simulink model "RmtAPP_DD1"  (R2016b)
settings: configuration reference "CodeGenConfigSet" (kept outside this file)
values from neighbouring files (symbols this model uses):
  RmtAPP_tiSRCHighDefDeb_C = Calibration.Parameter    [init_RmtAPP_DD1.m]    (also in init_RmtAPP_DD1_SIL.m = Simulink.Parameter)
  RmtAPP_tiSRCHighOKDeb_C = Calibration.Parameter    [init_RmtAPP_DD1.m]    (also in init_RmtAPP_DD1_SIL.m = Simulink.Parameter)
  RmtAPP_tiSRCLowDefDeb_C = Calibration.Parameter    [init_RmtAPP_DD1.m]    (also in init_RmtAPP_DD1_SIL.m = Simulink.Parameter)
  RmtAPP_tiSRCLowOKDeb_C = Calibration.Parameter    [init_RmtAPP_DD1.m]    (also in init_RmtAPP_DD1_SIL.m = Simulink.Parameter)
  RmtAPP_uRaw1Def_C = Calibration.Parameter    [init_RmtAPP_DD1.m]    (also in init_RmtAPP_DD1_SIL.m = Simulink.Parameter)
  RmtAPP_uRaw1SRCHigh_C = Calibration.Parameter    [init_RmtAPP_DD1.m]    (also in init_RmtAPP_DD1_SIL.m = Simulink.Parameter)
  RmtAPP_uRaw1SRCLow_C = Calibration.Parameter    [init_RmtAPP_DD1.m]    (also in init_RmtAPP_DD1_SIL.m = Simulink.Parameter)
undefined symbols (not defined in the file or in its folder): RmtAPP_DD1_DT
libraries: CXLib x6
settings Model: Creator=bianxuyin  LastModifiedBy=bianxuyin
settings ConfigSetRef: SourceLocation=Base Workspace

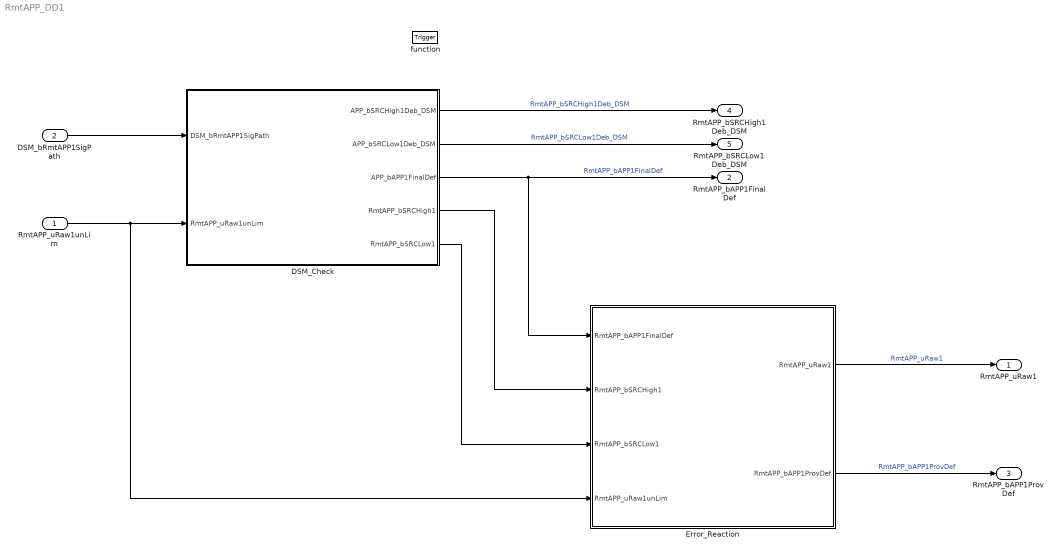
== system RmtAPP_DD1 ==
  RmtAPP_uRaw1unLim : Inport  Tag=mv  Description=Remote Acceleration pedal sensor 1 unlimited raw value  OutMin=0  OutMax=5000  OutDataTypeStr=Ad_mv
  DSM_bRmtAPP1SigPath : Inport  Description=status of FId_RmtAPP1SigPath  Port=2  OutMin=0  OutMax=1  OutDataTypeStr=boolean
  function : TriggerPort  TriggerType=function-call  VariantControl=Variant
  DSM_Check : Subsystem
  Error_Reaction : Subsystem
  RmtAPP_uRaw1 : Outport  Tag=mv  Description=Remote Acceleration Pedal Position D  OutMin=0  OutMax=5000  OutDataTypeStr=Ad_mv
  RmtAPP_bAPP1FinalDef : Outport  Description=Status Sensor 1 of the remote acceleration pedal finally defect  Port=2  OutMin=0  OutMax=1  OutDataTypeStr=boolean
  RmtAPP_bAPP1ProvDef : Outport  Description=Status Sensor 1 of the remote acceleration pedal temporary defect  Port=3  OutMin=0  OutMax=1  OutDataTypeStr=boolean
  RmtAPP_bSRCHigh1Deb_DSM : Outport  Description=Status debounced SRC-High error Sensor 1  Port=4  OutMin=0  OutMax=1  OutDataTypeStr=boolean
  RmtAPP_bSRCLow1Deb_DSM : Outport  Description=Status debounced SRC-Low error Sensor 1  Port=5  OutMin=0  OutMax=1  OutDataTypeStr=boolean
  wires:
  Error_Reaction/1(RmtAPP_uRaw1) -> RmtAPP_uRaw1/1  "RmtAPP_uRaw1"
  DSM_Check/3(APP_bAPP1FinalDef) -> Error_Reaction/1(RmtAPP_bAPP1FinalDef), RmtAPP_bAPP1FinalDef/1  "RmtAPP_bAPP1FinalDef"
  Error_Reaction/2(RmtAPP_bAPP1ProvDef) -> RmtAPP_bAPP1ProvDef/1  "RmtAPP_bAPP1ProvDef"
  DSM_Check/1(APP_bSRCHigh1Deb_DSM) -> RmtAPP_bSRCHigh1Deb_DSM/1  "RmtAPP_bSRCHigh1Deb_DSM"
  DSM_Check/2(APP_bSRCLow1Deb_DSM) -> RmtAPP_bSRCLow1Deb_DSM/1  "RmtAPP_bSRCLow1Deb_DSM"
  RmtAPP_uRaw1unLim/1 -> DSM_Check/2(RmtAPP_uRaw1unLim), Error_Reaction/4(RmtAPP_uRaw1unLim)
  DSM_bRmtAPP1SigPath/1 -> DSM_Check/1(DSM_bRmtAPP1SigPath)
  DSM_Check/4(RmtAPP_bSRCHigh1) -> Error_Reaction/2(RmtAPP_bSRCHigh1)
  DSM_Check/5(RmtAPP_bSRCLow1) -> Error_Reaction/3(RmtAPP_bSRCLow1)

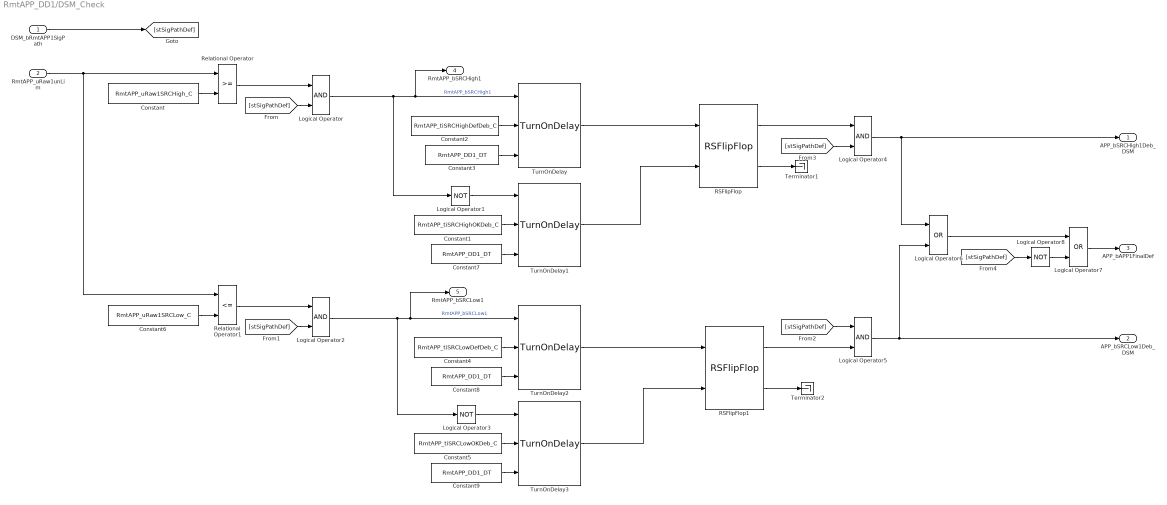
== system RmtAPP_DD1/DSM_Check ==
  DSM_bRmtAPP1SigPath : Inport  Description=status of FId_RmtAPP1SigPath  OutMin=0  OutMax=1  OutDataTypeStr=boolean
  RmtAPP_uRaw1unLim : Inport  Tag=mv  Description=Remote Acceleration pedal sensor 1 unlimited raw value  Port=2  OutMin=0  OutMax=5000  OutDataTypeStr=Ad_mv
  Constant : Constant  Value=RmtAPP_uRaw1SRCHigh_C
  Constant1 : Constant  Value=RmtAPP_tiSRCHighOKDeb_C
  Constant2 : Constant  Value=RmtAPP_tiSRCHighDefDeb_C
  Constant{3,7..9} (4 alike) : Constant  Value=RmtAPP_DD1_DT  OutDataTypeStr=Inherit: Inherit via back propagation
  Constant4 : Constant  Value=RmtAPP_tiSRCLowDefDeb_C
  Constant5 : Constant  Value=RmtAPP_tiSRCLowOKDeb_C
  Constant6 : Constant  Value=RmtAPP_uRaw1SRCLow_C
  Logical Operator{,2,4..5} (4 alike) : Logic  AllPortsSameDT=off  OutDataTypeStr=boolean
  Logical Operator1 : Logic  Operator=NOT  AllPortsSameDT=off  OutDataTypeStr=boolean
  Logical Operator3 : Logic  Operator=NOT  AllPortsSameDT=off  OutDataTypeStr=boolean
  Logical Operator6 : Logic  Operator=OR  AllPortsSameDT=off  OutDataTypeStr=boolean
  Logical Operator7 : Logic  Operator=OR  AllPortsSameDT=off  OutDataTypeStr=boolean
  Logical Operator8 : Logic  Operator=NOT  AllPortsSameDT=off  OutDataTypeStr=boolean
  RSFlipFlop : CXLib/RSFlipFlop
  RSFlipFlop1 : CXLib/RSFlipFlop
  Relational Operator : RelationalOperator  OutDataTypeStr=boolean  RndMeth=Simplest
  Relational Operator1 : RelationalOperator  Operator=<=  OutDataTypeStr=boolean  RndMeth=Simplest
  Terminator1 : Terminator
  Terminator2 : Terminator
  TurnOnDelay{,1..3} (4 alike) : CXLib/TurnOnDelay
  APP_bSRCHigh1Deb_DSM : Outport  Description=Status debounced SRC-High error Sensor 1  OutMin=0  OutMax=1  OutDataTypeStr=boolean
  APP_bSRCLow1Deb_DSM : Outport  Description=Status debounced SRC-Low error Sensor 1  Port=2  OutMin=0  OutMax=1  OutDataTypeStr=boolean
  APP_bAPP1FinalDef : Outport  Description=Status Sensor 1 of the acceleration pedal finally defect  Port=3  OutMin=0  OutMax=1  OutDataTypeStr=boolean
  RmtAPP_bSRCHigh1 : Outport  Tag=mv  Description=Remote Acceleration Pedal Position D  Port=4  OutMin=0  OutMax=1
  RmtAPP_bSRCLow1 : Outport  Tag=mv  Description=Remote Acceleration Pedal Position D  Port=5  OutMin=0  OutMax=1
  wires:
  DSM_bRmtAPP1SigPath/1 -> [stSigPathDef]
  RmtAPP_uRaw1unLim/1 -> Relational Operator1/1, Relational Operator/1
  Relational Operator/1 -> Logical Operator/1
  [stSigPathDef] -> Logical Operator/2
  Constant/1 -> Relational Operator/2
  Logical Operator/1 -> Logical Operator1/1, RmtAPP_bSRCHigh1/1, TurnOnDelay/1  "RmtAPP_bSRCHigh1"
  Logical Operator1/1 -> TurnOnDelay1/1
  Constant2/1 -> TurnOnDelay/2
  Constant3/1 -> TurnOnDelay/3
  Constant1/1 -> TurnOnDelay1/2
  Constant7/1 -> TurnOnDelay1/3
  Constant4/1 -> TurnOnDelay2/2
  Constant8/1 -> TurnOnDelay2/3
  Constant5/1 -> TurnOnDelay3/2
  Constant9/1 -> TurnOnDelay3/3
  Relational Operator1/1 -> Logical Operator2/1
  [stSigPathDef] -> Logical Operator2/2
  Constant6/1 -> Relational Operator1/2
  Logical Operator2/1 -> Logical Operator3/1, RmtAPP_bSRCLow1/1, TurnOnDelay2/1  "RmtAPP_bSRCLow1"
  Logical Operator3/1 -> TurnOnDelay3/1
  TurnOnDelay/1 -> RSFlipFlop/1
  TurnOnDelay3/1 -> RSFlipFlop1/2
  TurnOnDelay2/1 -> RSFlipFlop1/1
  TurnOnDelay1/1 -> RSFlipFlop/2
  RSFlipFlop1/1 -> Logical Operator5/2
  [stSigPathDef] -> Logical Operator5/1
  RSFlipFlop/1 -> Logical Operator4/1
  [stSigPathDef] -> Logical Operator4/2
  RSFlipFlop/2 -> Terminator1/1
  RSFlipFlop1/2 -> Terminator2/1
  Logical Operator5/1 -> Logical Operator6/2, APP_bSRCLow1Deb_DSM/1
  Logical Operator4/1 -> APP_bSRCHigh1Deb_DSM/1, Logical Operator6/1
  Logical Operator6/1 -> Logical Operator7/1
  [stSigPathDef] -> Logical Operator8/1
  Logical Operator8/1 -> Logical Operator7/2
  Logical Operator7/1 -> APP_bAPP1FinalDef/1

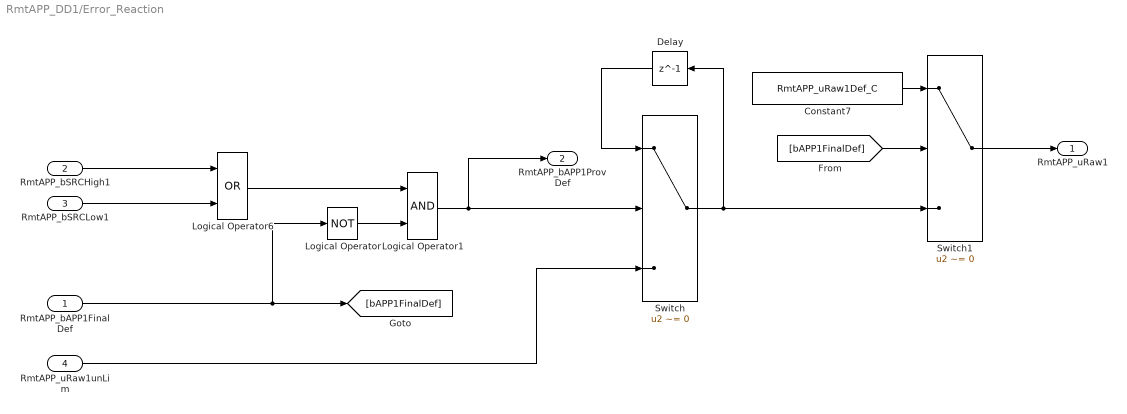
== system RmtAPP_DD1/Error_Reaction ==
  RmtAPP_bAPP1FinalDef : Inport
  RmtAPP_bSRCHigh1 : Inport  Port=2
  RmtAPP_bSRCLow1 : Inport  Port=3
  RmtAPP_uRaw1unLim : Inport  Port=4
  Constant7 : Constant  Value=RmtAPP_uRaw1Def_C
  Delay : Delay  DelayLength=1  InitialCondition=0
  Logical Operator : Logic  Operator=NOT  AllPortsSameDT=off  OutDataTypeStr=boolean
  Logical Operator1 : Logic  AllPortsSameDT=off  OutDataTypeStr=boolean
  Logical Operator6 : Logic  Operator=OR  AllPortsSameDT=off  OutDataTypeStr=boolean
  Switch : Switch  Criteria=u2 ~= 0
  Switch1 : Switch  Criteria=u2 ~= 0
  RmtAPP_uRaw1 : Outport  Tag=mv  Description=Acceleration Pedal Position D  OutMin=0  OutMax=5000  OutDataTypeStr=Ad_mv
  RmtAPP_bAPP1ProvDef : Outport  Tag=-  Description=Status Sensor 1 of the acceleration pedal temporary defect  Port=2  OutMin=0  OutMax=1  OutDataTypeStr=boolean
  wires:
  RmtAPP_bSRCHigh1/1 -> Logical Operator6/1
  RmtAPP_bSRCLow1/1 -> Logical Operator6/2
  Logical Operator6/1 -> Logical Operator1/1
  Logical Operator/1 -> Logical Operator1/2
  RmtAPP_bAPP1FinalDef/1 -> [bAPP1FinalDef], Logical Operator/1
  Logical Operator1/1 -> RmtAPP_bAPP1ProvDef/1, Switch/2
  RmtAPP_uRaw1unLim/1 -> Switch/3
  Switch/1 -> Delay/1, Switch1/3
  [bAPP1FinalDef] -> Switch1/2
  Constant7/1 -> Switch1/1
  Delay/1 -> Switch/1
  Switch1/1 -> RmtAPP_uRaw1/1
